simulink model "coordinate_transform_dcm"  (R2018a)
settings: Solver=VariableStepAuto  StartTime=0.0  StopTime=10.0  RelTol=1e-3
settings Model: Creator=lamy  LastModifiedBy=lamy

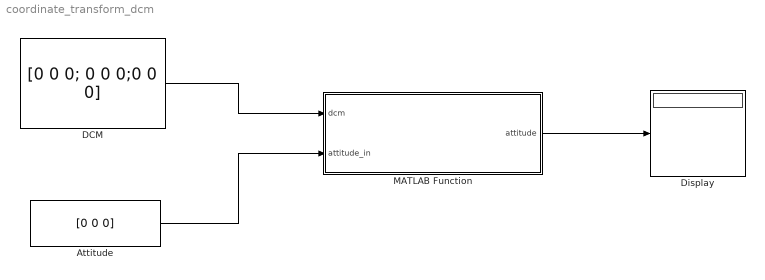
== system coordinate_transform_dcm ==
  Attitude : Constant  Value=[0 0 0]
  DCM : Constant  Value=[0 0 0; 0 0 0;0 0 0]
  Display : Display
  MATLAB Function : MATLAB Function  TreatAsAtomicUnit=on
  wires:
  DCM/1 -> MATLAB Function/1(dcm)
  Attitude/1 -> MATLAB Function/2(attitude_in)
  MATLAB Function/1(attitude) -> Display/1

== matlab function coordinate_transform_dcm/MATLAB Function ==
  data: dcm input; attitude output; attitude_in input
function attitude = coordinate_transform(dcm,attitude_in)
attitude = dcm*attitude_in;
